simulink model "nuri3s_PDG_DOB_final2"  (R2024b)
settings: Solver=VariableStepAuto  StartTime=0.0  StopTime=10  RelTol=1e-3
undefined symbols (not defined in the file): timepoints, waypoints
libraries: robotmaniplib x3, robotcorelib x1
settings Model: Creator=user  LastModifiedBy=leeyh

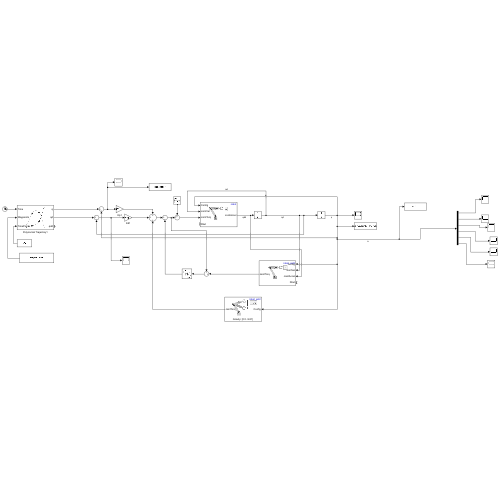
[thumbnail: Simulink's stored preview of the top-level diagram]
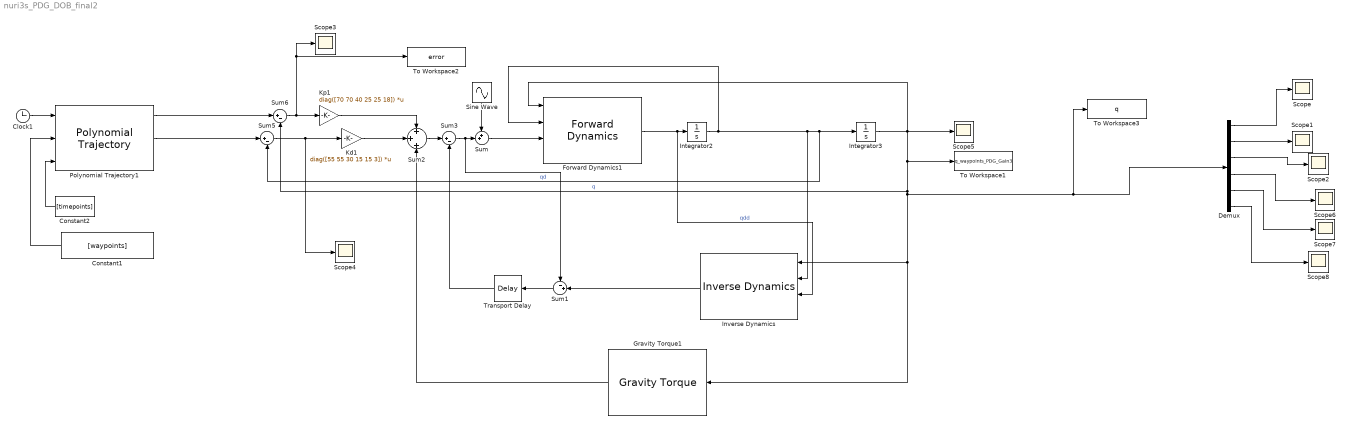
== system nuri3s_PDG_DOB_final2 ==
  Clock1 : Clock
  Constant1 : Constant  Value=[waypoints]
  Constant2 : Constant  Value=[timepoints]
  Demux : Demux  Outputs=6
  Forward Dynamics1 : robotmaniplib/Forward Dynamics  RigidBodyTree=robot  SimulateUsing=Interpreted execution
  Gravity Torque1 : robotmaniplib/Gravity Torque  RigidBodyTree=robot_est2  SimulateUsing=Interpreted execution
  Integrator2 : Integrator  InitialCondition=[0 0 -1.57 0 -1.57 0]
  Integrator3 : Integrator  InitialCondition=[0 0 -1.57 0 -1.57 0]
  Inverse Dynamics : robotmaniplib/Inverse Dynamics  RigidBodyTree=robot_est2  SimulateUsing=Interpreted execution
  Kd1 : Gain  Gain=diag([55 55 30 15 15 3])  Multiplication=Matrix(K*u)
  Kp1 : Gain  Gain=diag([70 70 40 25 25 18])  Multiplication=Matrix(K*u)
  Polynomial Trajectory1 : robotcorelib/Polynomial Trajectory  WaypointSource=External  Waypoints=[ 0, 2, 1, 5, 0; -1, 3, 1, 4, 4 ]  TimePoints=[ 0, 1, 2, 3, 4 ]  TimeInterval=[ 1, 4 ]  Method=Quintic Polynomial  ParameterSource=Internal  VelocityBoundaryCondition=zeros( 6, 100 )  AccelerationBoundaryCondition=zeros( 6, 100 )  SimulateUsing=Interpreted execution
  Scope{,1..8} (9 alike) : Scope
  Sine Wave : Sin  Amplitude=0.1  Frequency=10  SampleTime=0
  Sum : Sum  Inputs=++|
  Sum1 : Sum  Inputs=-+|
  Sum2 : Sum  Inputs=+|+|+
  Sum3 : Sum  Inputs=|+-
  Sum5 : Sum  Inputs=|+-
  Sum6 : Sum  Inputs=|+-
  To Workspace1 : ToWorkspace  VariableName=q_waypoints_PDG_Gain3  SampleTime=-1
  To Workspace2 : ToWorkspace  VariableName=error  SaveFormat=Structure With Time  SampleTime=-1
  To Workspace3 : ToWorkspace  VariableName=q  SaveFormat=Structure With Time  SampleTime=-1
  Transport Delay : TransportDelay  DelayTime=0.001
  wires:
  Gravity Torque1/1 -> Sum2/3
  Sum6/1 -> To Workspace2/1, Scope3/1, Kp1/1
  Integrator3/1 -> Forward Dynamics1/1, Scope5/1, To Workspace1/1, To Workspace3/1, Demux/1, Inverse Dynamics/1, Gravity Torque1/1, Sum6/2  "q"
  Integrator2/1 -> Inverse Dynamics/2, Integrator3/1, Sum5/2, Forward Dynamics1/2  "qd"
  Forward Dynamics1/1 -> Inverse Dynamics/3, Integrator2/1  "qdd"
  Sum5/1 -> Kd1/1, Scope4/1
  Polynomial Trajectory1/2 -> Sum5/1
  Polynomial Trajectory1/1 -> Sum6/1
  Constant1/1 -> Polynomial Trajectory1/2
  Constant2/1 -> Polynomial Trajectory1/3
  Clock1/1 -> Polynomial Trajectory1/1
  Demux/1 -> Scope/1
  Demux/2 -> Scope1/1
  Demux/3 -> Scope2/1
  Demux/4 -> Scope6/1
  Demux/5 -> Scope7/1
  Demux/6 -> Scope8/1
  Sum/1 -> Forward Dynamics1/3
  Sine Wave/1 -> Sum/1
  Inverse Dynamics/1 -> Sum1/2
  Sum1/1 -> Transport Delay/1
  Kd1/1 -> Sum2/2
  Kp1/1 -> Sum2/1
  Sum2/1 -> Sum3/1
  Transport Delay/1 -> Sum3/2
  Sum3/1 -> Sum1/1, Sum/2
